simulink model "control_filtro_dq_mod"  (R2017b)
settings: Solver=ode1  StartTime=0.0  StopTime=Tsim  FixedStep=Ts  MaxStep=1e-4  RelTol=1e-3
InitFcn:
  | GlobalParam
values from neighbouring files (symbols this model uses):
  APFon = 0.015    [GlobalParam.m]
  Cdc = 680e-6    (= 0.00068)    [GlobalParam.m]
  fc = 15000    [GlobalParam.m]
  fe = 50    [GlobalParam.m]
  Ideal = 1    [GlobalParam.m]
  Ki = 0.007    [GlobalParam.m]
  Kp = 0.006    [GlobalParam.m]
  Lf = 0.01    [GlobalParam.m]
  LL = 0.055462    [GlobalParam.m]
  nc = 3    [GlobalParam.m]
  Rf = 0.35    [GlobalParam.m]
  RL = 23.232    [GlobalParam.m]
  teta_a = 0    [GlobalParam.m]
  teta_b = 120    [GlobalParam.m]
  teta_c = -120    [GlobalParam.m]
  Tm = 1/fm    (= 6.66666666667e-05)    [GlobalParam.m]
  Ts = 10e-6    (= 1e-05)    [GlobalParam.m]
  Vdc = 62    [GlobalParam.m]
  Vs = 120*sqrt(2)    [GlobalParam.m]
libraries: powerlib x112, simulink x10, powerlib_extras x3, peTransforms x2, cstblocks x2, peSinusoidalMeasurement x1, powerlib_meascontrol x1
(part 2 of 2)

== system control_filtro_dq_mod/Convertidor multinivel CHB/Single-Phase CHB2/H-Bridge Driver2 ==
  si1 : Inport
  si3 : Inport  Port=2
  Logical Operator2 : Logic  Operator=NOT  AllPortsSameDT=off  OutDataTypeStr=boolean
  Logical Operator3 : Logic  Operator=NOT  AllPortsSameDT=off  OutDataTypeStr=boolean
  1 : Outport
  2 : Outport  Port=2
  3 : Outport  Port=3
  4 : Outport  Port=4
  wires:
  si3/1 -> 3/1, Logical Operator3/1
  si1/1 -> 1/1, Logical Operator2/1
  Logical Operator3/1 -> 4/1
  Logical Operator2/1 -> 2/1

== system control_filtro_dq_mod/Convertidor multinivel CHB/Single-Phase CHB2/H-Bridge Driver3 ==
  si1 : Inport
  si3 : Inport  Port=2
  Logical Operator2 : Logic  Operator=NOT  AllPortsSameDT=off  OutDataTypeStr=boolean
  Logical Operator3 : Logic  Operator=NOT  AllPortsSameDT=off  OutDataTypeStr=boolean
  1 : Outport
  2 : Outport  Port=2
  3 : Outport  Port=3
  4 : Outport  Port=4
  wires:
  si3/1 -> 3/1, Logical Operator3/1
  si1/1 -> 1/1, Logical Operator2/1
  Logical Operator3/1 -> 4/1
  Logical Operator2/1 -> 2/1

== system control_filtro_dq_mod/Convertidor multinivel CHB/Single-Phase CHB3/DC-Link1 ==
  Constant : Constant  Value=Ideal
  DC Capacitor : powerlib/Elements/Series RLC Branch  LConnTagsString=__new0  RConnTagsString=__new0  BranchType=C  Resistance=0.09  Inductance=0.002996  SetiL0=off  InitialCurrent=0  Capacitance=Cdc  Setx0=on  InitialVoltage=Vodc  Measurements=None
  DC Voltage Source : powerlib/Electrical Sources/DC Voltage Source  Amplitude=Vdc  Measurements=None
  Ideal Switch : powerlib/Power Electronics/Ideal Switch  Ron=0.001  Lon=0  IC=0  Rs=1e5  Cs=inf  Measurements=off
  Ideal Switch2 : powerlib/Power Electronics/Ideal Switch  Ron=0.001  Lon=0  IC=0  Rs=1e5  Cs=inf  Measurements=off
  Logical Operator2 : Logic  Operator=NOT  AllPortsSameDT=off  OutDataTypeStr=boolean
  Vcan3 : powerlib/Measurements/Voltage Measurement  PhasorSimulation=off  OutputType=Complex  PSBequivalent=0
  + : PMIOPort  Port=1  Side=Right
  - : PMIOPort  Port=2  Side=Right
  tag scope: Vccc1=global
  wires:
  Constant/1 -> Ideal Switch/1, Logical Operator2/1
  Logical Operator2/1 -> Ideal Switch2/1
  Vcan3/1 -> [Vccc1]
  connections:
  DC Capacitor/LConn1 -- Ideal Switch2/LConn1
  Ideal Switch/RConn1 -- Ideal Switch2/RConn1 -- Vcan3/LConn1 -- +/RConn1
  DC Voltage Source/RConn1 -- Ideal Switch/LConn1
  -/RConn1 -- Vcan3/LConn2 -- DC Voltage Source/LConn1 -- DC Capacitor/RConn1

== system control_filtro_dq_mod/Convertidor multinivel CHB/Single-Phase CHB3/DC-Link2 ==
  Constant : Constant  Value=Ideal
  DC Capacitor : powerlib/Elements/Series RLC Branch  LConnTagsString=__new0  RConnTagsString=__new0  BranchType=C  Resistance=0.09  Inductance=0.002996  SetiL0=off  InitialCurrent=0  Capacitance=Cdc  Setx0=on  InitialVoltage=Vodc  Measurements=None
  DC Voltage Source : powerlib/Electrical Sources/DC Voltage Source  Amplitude=Vdc  Measurements=None
  Ideal Switch : powerlib/Power Electronics/Ideal Switch  Ron=0.001  Lon=0  IC=0  Rs=1e5  Cs=inf  Measurements=off
  Ideal Switch2 : powerlib/Power Electronics/Ideal Switch  Ron=0.001  Lon=0  IC=0  Rs=1e5  Cs=inf  Measurements=off
  Logical Operator2 : Logic  Operator=NOT  AllPortsSameDT=off  OutDataTypeStr=boolean
  Vcan3 : powerlib/Measurements/Voltage Measurement  PhasorSimulation=off  OutputType=Complex  PSBequivalent=0
  + : PMIOPort  Port=1  Side=Right
  - : PMIOPort  Port=2  Side=Right
  tag scope: Vccc2=global
  wires:
  Constant/1 -> Ideal Switch/1, Logical Operator2/1
  Logical Operator2/1 -> Ideal Switch2/1
  Vcan3/1 -> [Vccc2]
  connections:
  Ideal Switch/RConn1 -- Ideal Switch2/RConn1 -- Vcan3/LConn1 -- +/RConn1
  DC Voltage Source/RConn1 -- Ideal Switch/LConn1
  -/RConn1 -- DC Capacitor/RConn1 -- DC Voltage Source/LConn1 -- Vcan3/LConn2
  Ideal Switch2/LConn1 -- DC Capacitor/LConn1

== system control_filtro_dq_mod/Convertidor multinivel CHB/Single-Phase CHB3/DC-Link3 ==
  Constant : Constant  Value=Ideal
  DC Capacitor : powerlib/Elements/Series RLC Branch  LConnTagsString=__new0  RConnTagsString=__new0  BranchType=C  Resistance=0.09  Inductance=0.002996  SetiL0=off  InitialCurrent=0  Capacitance=Cdc  Setx0=on  InitialVoltage=Vodc  Measurements=None
  DC Voltage Source : powerlib/Electrical Sources/DC Voltage Source  Amplitude=Vdc  Measurements=None
  Ideal Switch : powerlib/Power Electronics/Ideal Switch  Ron=0.001  Lon=0  IC=0  Rs=1e5  Cs=inf  Measurements=off
  Ideal Switch2 : powerlib/Power Electronics/Ideal Switch  Ron=0.001  Lon=0  IC=0  Rs=1e5  Cs=inf  Measurements=off
  Logical Operator2 : Logic  Operator=NOT  AllPortsSameDT=off  OutDataTypeStr=boolean
  Vcan3 : powerlib/Measurements/Voltage Measurement  PhasorSimulation=off  OutputType=Complex  PSBequivalent=0
  + : PMIOPort  Port=1  Side=Right
  - : PMIOPort  Port=2  Side=Right
  tag scope: Vccc3=global
  wires:
  Constant/1 -> Ideal Switch/1, Logical Operator2/1
  Logical Operator2/1 -> Ideal Switch2/1
  Vcan3/1 -> [Vccc3]
  connections:
  Ideal Switch/RConn1 -- Ideal Switch2/RConn1 -- Vcan3/LConn1 -- +/RConn1
  DC Voltage Source/RConn1 -- Ideal Switch/LConn1
  -/RConn1 -- Vcan3/LConn2 -- DC Capacitor/RConn1 -- DC Voltage Source/LConn1
  Ideal Switch2/LConn1 -- DC Capacitor/LConn1

== system control_filtro_dq_mod/Convertidor multinivel CHB/Single-Phase CHB3/H-Bridge Cell1 ==
  si1 : Inport
  si2 : Inport  Port=2
  si3 : Inport  Port=3
  si4 : Inport  Port=4
  IGBT/Diode{1..4} (4 alike) : powerlib/Power Electronics/IGBT//Diode  Ron=Ron  Rs=Rs  Cs=Cs  Measurements=off
  DC+ : PMIOPort  Port=1  Side=Right
  DC- : PMIOPort  Port=2  Side=Right
  + : PMIOPort  Port=3  Side=Right
  - : PMIOPort  Port=4  Side=Right
  wires:
  si4/1 -> IGBT/Diode4/1
  si2/1 -> IGBT/Diode2/1
  si3/1 -> IGBT/Diode3/1
  si1/1 -> IGBT/Diode1/1
  connections:
  IGBT/Diode3/RConn1 -- -/RConn1 -- IGBT/Diode4/LConn1
  IGBT/Diode2/RConn1 -- DC-/RConn1 -- IGBT/Diode4/RConn1
  IGBT/Diode1/RConn1 -- +/RConn1 -- IGBT/Diode2/LConn1
  IGBT/Diode1/LConn1 -- IGBT/Diode3/LConn1 -- DC+/RConn1

== system control_filtro_dq_mod/Convertidor multinivel CHB/Single-Phase CHB3/H-Bridge Cell2 ==
  si1 : Inport
  si2 : Inport  Port=2
  si3 : Inport  Port=3
  si4 : Inport  Port=4
  IGBT/Diode{1..4} (4 alike) : powerlib/Power Electronics/IGBT//Diode  Ron=Ron  Rs=Rs  Cs=Cs  Measurements=off
  DC+ : PMIOPort  Port=1  Side=Right
  DC- : PMIOPort  Port=2  Side=Right
  + : PMIOPort  Port=3  Side=Right
  - : PMIOPort  Port=4  Side=Right
  wires:
  si4/1 -> IGBT/Diode4/1
  si2/1 -> IGBT/Diode2/1
  si3/1 -> IGBT/Diode3/1
  si1/1 -> IGBT/Diode1/1
  connections:
  IGBT/Diode3/RConn1 -- IGBT/Diode4/LConn1 -- -/RConn1
  IGBT/Diode2/RConn1 -- IGBT/Diode4/RConn1 -- DC-/RConn1
  IGBT/Diode1/RConn1 -- IGBT/Diode2/LConn1 -- +/RConn1
  IGBT/Diode1/LConn1 -- IGBT/Diode3/LConn1 -- DC+/RConn1

== system control_filtro_dq_mod/Convertidor multinivel CHB/Single-Phase CHB3/H-Bridge Cell3 ==
  si1 : Inport
  si2 : Inport  Port=2
  si3 : Inport  Port=3
  si4 : Inport  Port=4
  IGBT/Diode{1..4} (4 alike) : powerlib/Power Electronics/IGBT//Diode  Ron=Ron  Rs=Rs  Cs=Cs  Measurements=off
  DC+ : PMIOPort  Port=1  Side=Right
  DC- : PMIOPort  Port=2  Side=Right
  + : PMIOPort  Port=3  Side=Right
  - : PMIOPort  Port=4  Side=Right
  wires:
  si4/1 -> IGBT/Diode4/1
  si2/1 -> IGBT/Diode2/1
  si3/1 -> IGBT/Diode3/1
  si1/1 -> IGBT/Diode1/1
  connections:
  IGBT/Diode3/RConn1 -- IGBT/Diode4/LConn1 -- -/RConn1
  IGBT/Diode2/RConn1 -- IGBT/Diode4/RConn1 -- DC-/RConn1
  IGBT/Diode1/RConn1 -- IGBT/Diode2/LConn1 -- +/RConn1
  IGBT/Diode1/LConn1 -- IGBT/Diode3/LConn1 -- DC+/RConn1

== system control_filtro_dq_mod/Convertidor multinivel CHB/Single-Phase CHB3/H-Bridge Driver1 ==
  si1 : Inport
  si3 : Inport  Port=2
  Logical Operator2 : Logic  Operator=NOT  AllPortsSameDT=off  OutDataTypeStr=boolean
  Logical Operator3 : Logic  Operator=NOT  AllPortsSameDT=off  OutDataTypeStr=boolean
  1 : Outport
  2 : Outport  Port=2
  3 : Outport  Port=3
  4 : Outport  Port=4
  wires:
  si3/1 -> 3/1, Logical Operator3/1
  si1/1 -> 1/1, Logical Operator2/1
  Logical Operator3/1 -> 4/1
  Logical Operator2/1 -> 2/1

== system control_filtro_dq_mod/Convertidor multinivel CHB/Single-Phase CHB3/H-Bridge Driver2 ==
  si1 : Inport
  si3 : Inport  Port=2
  Logical Operator2 : Logic  Operator=NOT  AllPortsSameDT=off  OutDataTypeStr=boolean
  Logical Operator3 : Logic  Operator=NOT  AllPortsSameDT=off  OutDataTypeStr=boolean
  1 : Outport
  2 : Outport  Port=2
  3 : Outport  Port=3
  4 : Outport  Port=4
  wires:
  si3/1 -> 3/1, Logical Operator3/1
  si1/1 -> 1/1, Logical Operator2/1
  Logical Operator3/1 -> 4/1
  Logical Operator2/1 -> 2/1

== system control_filtro_dq_mod/Convertidor multinivel CHB/Single-Phase CHB3/H-Bridge Driver3 ==
  si1 : Inport
  si3 : Inport  Port=2
  Logical Operator2 : Logic  Operator=NOT  AllPortsSameDT=off  OutDataTypeStr=boolean
  Logical Operator3 : Logic  Operator=NOT  AllPortsSameDT=off  OutDataTypeStr=boolean
  1 : Outport
  2 : Outport  Port=2
  3 : Outport  Port=3
  4 : Outport  Port=4
  wires:
  si3/1 -> 3/1, Logical Operator3/1
  si1/1 -> 1/1, Logical Operator2/1
  Logical Operator3/1 -> 4/1
  Logical Operator2/1 -> 2/1
